simulink model "excercise1_tf_ex4"  (R2023b)
settings: Solver=VariableStepAuto  StartTime=0.0  StopTime=0.3  RelTol=1e-3
undefined symbols (not defined in the file): C, R
settings Model: Creator=elliot  LastModifiedBy=elliot

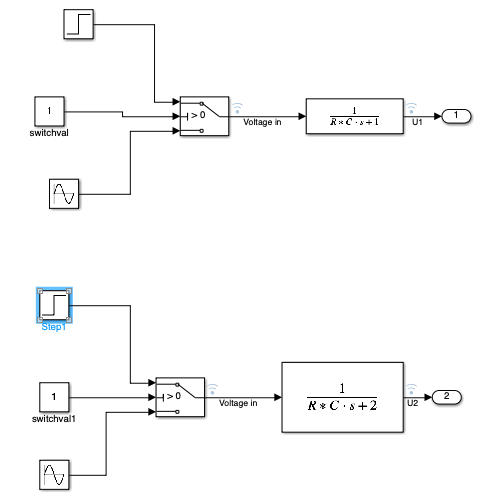
[thumbnail: Simulink's stored preview of the top-level diagram]
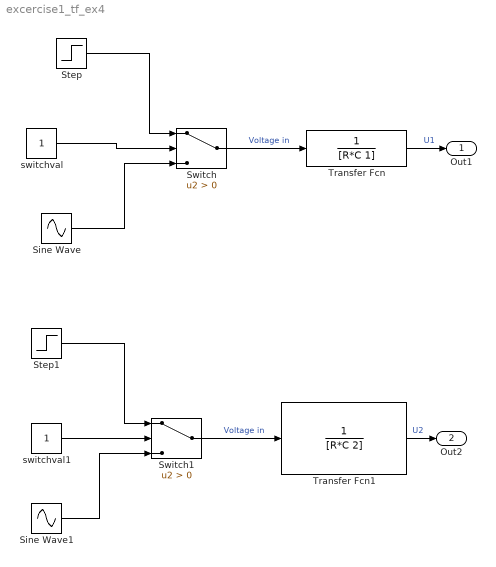
== system excercise1_tf_ex4 ==
  Sine Wave : Sin  Frequency=10  SampleTime=0
  Sine Wave1 : Sin  Frequency=10  SampleTime=0
  Step : Step  Time=0  After=12  SampleTime=0
  Step1 : Step  Time=0.2  After=12  SampleTime=0
  Switch : Switch  Criteria=u2 > Threshold  SaturateOnIntegerOverflow=off  InputSameDT=off
  Switch1 : Switch  Criteria=u2 > Threshold  SaturateOnIntegerOverflow=off  InputSameDT=off
  Transfer Fcn : TransferFcn  Denominator=[R*C 1]
  Transfer Fcn1 : TransferFcn  Denominator=[R*C 2]
  switchval : Constant
  switchval1 : Constant
  Out1 : Outport
  Out2 : Outport  Port=2
  wires:
  Step1/1 -> Switch1/1
  Switch1/1 -> Transfer Fcn1/1  "Voltage in"
  Step/1 -> Switch/1
  switchval/1 -> Switch/2
  Switch/1 -> Transfer Fcn/1  "Voltage in"
  Sine Wave/1 -> Switch/3
  Sine Wave1/1 -> Switch1/3
  switchval1/1 -> Switch1/2
  Transfer Fcn1/1 -> Out2/1  "U2"
  Transfer Fcn/1 -> Out1/1  "U1"
